simulink model "manipulator_controller"  (R2020b)
settings: Solver=VariableStepAuto  StartTime=0.0  StopTime=10.0  RelTol=1e-3
undefined symbols (not defined in the file or in its folder): X, Y, Z
libraries: sm_lib x46, nesl_utility x24, eeGeneralControl x12, pid_lib x11
(part 3 of 3)

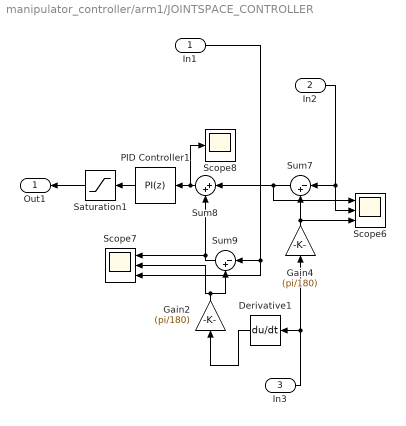
== system manipulator_controller/arm1/JOINTSPACE_CONTROLLER ==
  In1 : Inport
  In2 : Inport  Port=2
  In3 : Inport  Port=3
  Derivative1 : Derivative
  Gain2 : Gain  Gain=(pi/180)
  Gain4 : Gain  Gain=(pi/180)
  PID Controller1 : pid_lib/PID Controller  Controller=PI  Form=Parallel  TimeDomain=Discrete-time  UseExternalTs=off  SampleTime=.001  IntegratorMethod=Forward Euler  FilterMethod=Forward Euler  ControllerParametersSource=internal  P=1000  I=100  D=0  UseFilter=on  N=10  TunerSelectOption=Transfer Function Based (PID Tuner App)  InitialConditionSource=internal  InitialConditionForIntegrator=0  InitialConditionForFilter=0  DifferentiatorICPrevScaledInput=0  ExternalReset=none  TrackingMode=off  Kt=1  LimitOutput=off  SatLimitsSource=internal  UpperSaturationLimit=inf  LowerSaturationLimit=-inf  LinearizeAsGain=on  AntiWindupMode=none  Kb=1  POutMin=[]  POutMax=[]  IOutMin=[]  IOutMax=[]  DOutMin=[]  DOutMax=[]  NOutMin=[]  NOutMax=[]  SumOutMin=[]  SumOutMax=[]  SaturationOutMin=[]  SaturationOutMax=[]  PParamMin=[]  PParamMax=[]  IParamMin=[]  IParamMax=[]  DParamMin=[]  DParamMax=[]  NParamMin=[]  NParamMax=[]  KbParamMin=[]  KbParamMax=[]  KtParamMin=[]  KtParamMax=[]  KbOutMin=[]  KbOutMax=[]  KtOutMin=[]  KtOutMax=[]  IntegratorOutMin=[]  IntegratorOutMax=[]  FilterOutMin=[]  FilterOutMax=[]  SumI1OutMin=[]  SumI1OutMax=[]  SumI2OutMin=[]  SumI2OutMax=[]  SumI3OutMin=[]  SumI3OutMax=[]  SumI4OutMin=[]  SumI4OutMax=[]  SumDOutMin=[]  SumDOutMax=[]  DifferentiatorOutMin=[]  DifferentiatorOutMax=[]  FilterDiffOutCoefMin=[]  FilterDiffOutCoefMax=[]  ReciprocalOutMin=[]  ReciprocalOutMax=[]  SumDenOutMin=[]  SumDenOutMax=[]  SumNumOutMin=[]  SumNumOutMax=[]  DivideOutMin=[]  DivideOutMax=[]  UdiffTsProdOutMin=[]  UdiffTsProdOutMax=[]  NTsProdOutMin=[]  NTsProdOutMax=[]  UintegralTsProdOutMin=[]  UintegralTsProdOutMax=[]  UngainTsProdOutMin=[]  UngainTsProdOutMax=[]  IntegratorContinuousStateAttributes=''  IntegratorStateMustResolveToSignalObject=off  IntegratorRTWStateStorageClass=Auto  FilterContinuousStateAttributes=''  FilterStateMustResolveToSignalObject=off  FilterRTWStateStorageClass=Auto  ParallelPVariant=InternalParameters  IdealPVariant=Disabled  IVariant=InternalParameters  DVariant=Disabled  IntegratorVariant=Discrete  SatVariant=Disabled  AWVariant=Passthrough  PCopyVariant=Disabled  TRVariant=Disabled  FdbkBlocksVariant=Forward  IdealPFdbkVariant=Disabled  SatFdbkVariant=Disabled  DerivativeFilterVariant=Disabled  NVariant=Disabled  NCopyVariant=Disabled_SignalSpec  FilterICVariant=Disabled  IntegratorICVariant=InternalICs  ExternalResetVariant=Disabled  TRSumVariant=Passthrough  SumFdbkVariant=Disabled  SumVariant=Sum_PI  TsampFilterVariant=InternalTs  TsampNgainVariant=Passthrough  TsampIntegralVariant=Passthrough  ExternalSaturationOutDataTypeStr=Inherit: Same as second input
  Saturation1 : Saturate  UpperLimit=50  LowerLimit=-50
  Scope6 : Scope  NumInputPorts=3
  Scope7 : Scope  NumInputPorts=3
  Scope8 : Scope
  Sum7 : Sum  Inputs=|-+
  Sum8 : Sum  Inputs=|++
  Sum9 : Sum  Inputs=|-+
  Out1 : Outport
  wires:
  Sum9/1 -> Sum8/2, Scope7/1
  Sum7/1 -> Scope6/1, Sum8/1
  Gain2/1 -> Scope7/2, Sum9/2
  Gain4/1 -> Sum7/2, Scope6/3
  In2/1 -> Scope6/2, Sum7/1
  In3/1 -> Derivative1/1, Gain4/1
  In1/1 -> Scope7/3, Sum9/1
  Sum8/1 -> Scope8/1, PID Controller1/1
  PID Controller1/1 -> Saturation1/1
  Derivative1/1 -> Gain2/1
  Saturation1/1 -> Out1/1

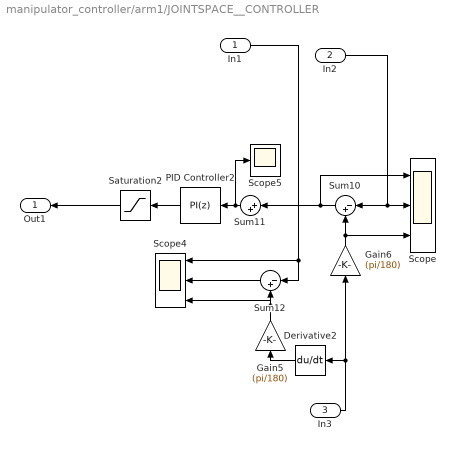
== system manipulator_controller/arm1/JOINTSPACE__CONTROLLER ==
  In1 : Inport
  In2 : Inport  Port=2
  In3 : Inport  Port=3
  Derivative2 : Derivative
  Gain5 : Gain  Gain=(pi/180)
  Gain6 : Gain  Gain=(pi/180)
  PID Controller2 : pid_lib/PID Controller  Controller=PI  Form=Parallel  TimeDomain=Discrete-time  UseExternalTs=off  SampleTime=.001  IntegratorMethod=Forward Euler  FilterMethod=Forward Euler  ControllerParametersSource=internal  P=300  I=30  D=0  UseFilter=on  N=10  TunerSelectOption=Transfer Function Based (PID Tuner App)  InitialConditionSource=internal  InitialConditionForIntegrator=0  InitialConditionForFilter=0  DifferentiatorICPrevScaledInput=0  ExternalReset=none  TrackingMode=off  Kt=1  LimitOutput=off  SatLimitsSource=internal  UpperSaturationLimit=inf  LowerSaturationLimit=-inf  LinearizeAsGain=on  AntiWindupMode=none  Kb=1  POutMin=[]  POutMax=[]  IOutMin=[]  IOutMax=[]  DOutMin=[]  DOutMax=[]  NOutMin=[]  NOutMax=[]  SumOutMin=[]  SumOutMax=[]  SaturationOutMin=[]  SaturationOutMax=[]  PParamMin=[]  PParamMax=[]  IParamMin=[]  IParamMax=[]  DParamMin=[]  DParamMax=[]  NParamMin=[]  NParamMax=[]  KbParamMin=[]  KbParamMax=[]  KtParamMin=[]  KtParamMax=[]  KbOutMin=[]  KbOutMax=[]  KtOutMin=[]  KtOutMax=[]  IntegratorOutMin=[]  IntegratorOutMax=[]  FilterOutMin=[]  FilterOutMax=[]  SumI1OutMin=[]  SumI1OutMax=[]  SumI2OutMin=[]  SumI2OutMax=[]  SumI3OutMin=[]  SumI3OutMax=[]  SumI4OutMin=[]  SumI4OutMax=[]  SumDOutMin=[]  SumDOutMax=[]  DifferentiatorOutMin=[]  DifferentiatorOutMax=[]  FilterDiffOutCoefMin=[]  FilterDiffOutCoefMax=[]  ReciprocalOutMin=[]  ReciprocalOutMax=[]  SumDenOutMin=[]  SumDenOutMax=[]  SumNumOutMin=[]  SumNumOutMax=[]  DivideOutMin=[]  DivideOutMax=[]  UdiffTsProdOutMin=[]  UdiffTsProdOutMax=[]  NTsProdOutMin=[]  NTsProdOutMax=[]  UintegralTsProdOutMin=[]  UintegralTsProdOutMax=[]  UngainTsProdOutMin=[]  UngainTsProdOutMax=[]  IntegratorContinuousStateAttributes=''  IntegratorStateMustResolveToSignalObject=off  IntegratorRTWStateStorageClass=Auto  FilterContinuousStateAttributes=''  FilterStateMustResolveToSignalObject=off  FilterRTWStateStorageClass=Auto  ParallelPVariant=InternalParameters  IdealPVariant=Disabled  IVariant=InternalParameters  DVariant=Disabled  IntegratorVariant=Discrete  SatVariant=Disabled  AWVariant=Passthrough  PCopyVariant=Disabled  TRVariant=Disabled  FdbkBlocksVariant=Forward  IdealPFdbkVariant=Disabled  SatFdbkVariant=Disabled  DerivativeFilterVariant=Disabled  NVariant=Disabled  NCopyVariant=Disabled_SignalSpec  FilterICVariant=Disabled  IntegratorICVariant=InternalICs  ExternalResetVariant=Disabled  TRSumVariant=Passthrough  SumFdbkVariant=Disabled  SumVariant=Sum_PI  TsampFilterVariant=InternalTs  TsampNgainVariant=Passthrough  TsampIntegralVariant=Passthrough  ExternalSaturationOutDataTypeStr=Inherit: Same as second input
  Saturation2 : Saturate  UpperLimit=50  LowerLimit=-50
  Scope : Scope  NumInputPorts=3
  Scope4 : Scope  NumInputPorts=3
  Scope5 : Scope
  Sum10 : Sum  Inputs=|-+
  Sum11 : Sum  Inputs=|++
  Sum12 : Sum  Inputs=|-+
  Out1 : Outport
  wires:
  Sum12/1 -> Scope4/2
  Derivative2/1 -> Gain5/1
  Gain6/1 -> Sum10/2, Scope/3
  In3/1 -> Gain6/1, Derivative2/1
  Sum10/1 -> Sum11/1, Scope/1
  In2/1 -> Sum10/1, Scope/2
  Saturation2/1 -> Out1/1
  PID Controller2/1 -> Saturation2/1
  In1/1 -> Scope4/1, Sum12/1
  Sum11/1 -> Scope5/1, PID Controller2/1
  Gain5/1 -> Sum12/2, Scope4/3

== matlab function manipulator_controller/arm1/FEEDFORWARD_GRAVITY EFFECTS/MATLAB Function3 ==
  data: Theta1 input; Theta2 input; alfa input; T1 output; r input
function T1 = fcn(Theta1, Theta2,alfa,r)
%int m = 1;         % mass of each block m = 1 Kg
%int L = 1;         % length of each block L = 1 m 
%int g = 9.80665;   % gravitional const g 
%int x1 = sin(Theta1) + (sin(Theta1 + Theta2))/2 ;
%int y1 = cos(Theta1) + (cos(Theta1 + Theta2))/2 ;
%int x2 = sin(Theta1) + sin(Theta1 + Theta2) + sin(Theta1 + Theta2 + Theta3)/2 ;
%int y2 = cos(Theta1) + cos(Theta1 + Theta2) + cos(Theta1 + Theta2 + Theta3)/2 ;

T1 = -9.80665*(sin(Theta1 + Theta2)/2 + r*sin(alfa) );

== matlab function manipulator_controller/arm1/FEEDFORWARD_GRAVITY EFFECTS/MATLAB Function4 ==
  data: theta1 input; theta2 input; theta3 input; y output
function y = fcn(theta1,theta2,theta3)

y = 1.2*cos(theta1+theta2+theta3)*.5*10;
end

== matlab function manipulator_controller/arm/MAIN_FUNCTION1 ==
  data: Theta1 input; Theta11 output; Theta2 input; Theta3 input; alpha1 output; r1 output; alpa2 output; r2 output
function [Theta11, alpha1, r1, alpa2, r2]= fcn(Theta1, Theta2, Theta3)

Theta11 = Theta1;
alpha1 = atan((2*sin(Theta1) + sin(Theta1 + Theta2))/(2*cos(Theta1) + cos(Theta1 + Theta2)));
r1 = sqrt((sin(Theta1) + (sin(Theta1 + Theta2))/2)^2  + (cos(Theta1) + (cos(Theta1 + Theta2))/2)^2);
alpa2 = atan((2*sin(Theta1) + 2*sin(Theta1 + Theta2) + sin(Theta1 + Theta2 + Theta3))/(2*cos(Theta1) + 2*cos(Theta1 + Theta2) + cos(Theta1 + Theta2 + Theta3)));
r2 = sqrt((sin(Theta1) + sin(Theta1 + Theta2) + sin(Theta1 + Theta2 + Theta3)/2)^2  +  ( cos(Theta1) + cos(Theta1 + Theta2) + cos(Theta1 + Theta2 + Theta3)/2)^2 );

== matlab function manipulator_controller/arm/JOINT1_FUNCTION ==
  data: Theta1 input; alpa1 input; r1 input; T1 output; alpa2 input; r2 input
function T1 = fcn(Theta1, alpa1,r1, alpa2,r2)
%int m = 1;         % mass of each block m = 1 Kg
%int L = 1;         % length of each block L = 1 m 
%int g = 9.80665;   % gravitional const g 
%int x1 = sin(Theta1) + (sin(Theta1 + Theta2))/2 ;
%int y1 = cos(Theta1) + (cos(Theta1 + Theta2))/2 ;
%int x2 = sin(Theta1) + sin(Theta1 + Theta2) + sin(Theta1 + Theta2 + Theta3)/2 ;
%int y2 = cos(Theta1) + cos(Theta1 + Theta2) + cos(Theta1 + Theta2 + Theta3)/2 ;

T1 = -9.80665*(sin(Theta1)/2 + r1*sin(alpa1) + r2*sin(alpa2) );

== matlab function manipulator_controller/arm/MATLAB Function2 ==
  data: Theta1 input; Theta11 output; Theta2 input; Theta3 input; Theta22 output; alfa output; r output
function [Theta11,Theta22,alfa,r]= fcn(Theta1, Theta2, Theta3)

Theta11 = Theta1;
Theta22 = Theta2;
alfa = atan(( 2*sin(Theta1 + Theta2) + sin(Theta1 + Theta2 + Theta3))/( 2*cos(Theta1 + Theta2) + cos(Theta1 + Theta2 + Theta3)));
r = sqrt(( sin(Theta1 + Theta2) + sin(Theta1 + Theta2 + Theta3)/2)^2  +  ( cos(Theta1 + Theta2) + cos(Theta1 + Theta2 + Theta3)/2)^2 );

== matlab function manipulator_controller/arm/MATLAB Function3 ==
  data: Theta1 input; Theta2 input; alfa input; T1 output; r input
function T1 = fcn(Theta1, Theta2,alfa,r)
%int m = 1;         % mass of each block m = 1 Kg
%int L = 1;         % length of each block L = 1 m 
%int g = 9.80665;   % gravitional const g 
%int x1 = sin(Theta1) + (sin(Theta1 + Theta2))/2 ;
%int y1 = cos(Theta1) + (cos(Theta1 + Theta2))/2 ;
%int x2 = sin(Theta1) + sin(Theta1 + Theta2) + sin(Theta1 + Theta2 + Theta3)/2 ;
%int y2 = cos(Theta1) + cos(Theta1 + Theta2) + cos(Theta1 + Theta2 + Theta3)/2 ;

T1 = -9.80665*(sin(Theta1 + Theta2)/2 + r*sin(alfa) );

== matlab function manipulator_controller/arm/JOINT3_FUNCTION ==
  data: theta1 input; theta2 input; theta3 input; y output
function y = fcn(theta1,theta2,theta3)

y = 1.2*cos(theta1+theta2+theta3)*.5*10;
end

== matlab function manipulator_controller/arm1/FEEDFORWARD_GRAVITY EFFECTS/MATLAB Function ==
  data: Theta1 input; alpa1 input; r1 input; T1 output; alpa2 input; r2 input
function T1 = fcn(Theta1, alpa1,r1, alpa2,r2)
%int m = 1;         % mass of each block m = 1 Kg
%int L = 1;         % length of each block L = 1 m 
%int g = 9.80665;   % gravitional const g 
%int x1 = sin(Theta1) + (sin(Theta1 + Theta2))/2 ;
%int y1 = cos(Theta1) + (cos(Theta1 + Theta2))/2 ;
%int x2 = sin(Theta1) + sin(Theta1 + Theta2) + sin(Theta1 + Theta2 + Theta3)/2 ;
%int y2 = cos(Theta1) + cos(Theta1 + Theta2) + cos(Theta1 + Theta2 + Theta3)/2 ;

T1 = -9.80665*(sin(Theta1)/2 + r1*sin(alpa1) + r2*sin(alpa2) );

== matlab function manipulator_controller/arm1/FEEDFORWARD_GRAVITY EFFECTS/MATLAB Function1 ==
  data: Theta1 input; Theta11 output; Theta2 input; Theta3 input; alpha1 output; r1 output; alpa2 output; r2 output
function [Theta11, alpha1, r1, alpa2, r2]= fcn(Theta1, Theta2, Theta3)

Theta11 = Theta1;
alpha1 = atan((2*sin(Theta1) + sin(Theta1 + Theta2))/(2*cos(Theta1) + cos(Theta1 + Theta2)));
r1 = sqrt((sin(Theta1) + (sin(Theta1 + Theta2))/2)^2  + (cos(Theta1) + (cos(Theta1 + Theta2))/2)^2);
alpa2 = atan((2*sin(Theta1) + 2*sin(Theta1 + Theta2) + sin(Theta1 + Theta2 + Theta3))/(2*cos(Theta1) + 2*cos(Theta1 + Theta2) + cos(Theta1 + Theta2 + Theta3)));
r2 = sqrt((sin(Theta1) + sin(Theta1 + Theta2) + sin(Theta1 + Theta2 + Theta3)/2)^2  +  ( cos(Theta1) + cos(Theta1 + Theta2) + cos(Theta1 + Theta2 + Theta3)/2)^2 );

== matlab function manipulator_controller/arm1/FEEDFORWARD_GRAVITY EFFECTS/MATLAB Function2 ==
  data: Theta1 input; Theta11 output; Theta2 input; Theta3 input; Theta22 output; alfa output; r output
function [Theta11,Theta22,alfa,r]= fcn(Theta1, Theta2, Theta3)

Theta11 = Theta1;
Theta22 = Theta2;
alfa = atan(( 2*sin(Theta1 + Theta2) + sin(Theta1 + Theta2 + Theta3))/( 2*cos(Theta1 + Theta2) + cos(Theta1 + Theta2 + Theta3)));
r = sqrt(( sin(Theta1 + Theta2) + sin(Theta1 + Theta2 + Theta3)/2)^2  +  ( cos(Theta1 + Theta2) + cos(Theta1 + Theta2 + Theta3)/2)^2 );
